simulink model "questao1lcsd3"  (R2026a)
settings: Solver=VariableStepAuto  MaxStep=1e-3
settings Model: Creator=shumy  LastModifiedBy=shumy

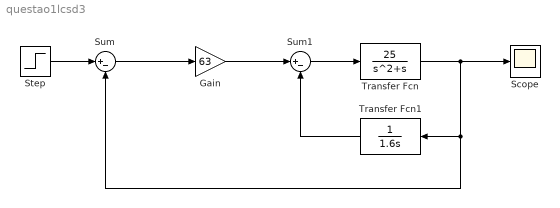
== system questao1lcsd3 ==
  Gain : Gain  Gain=63
  Scope : Scope
      settings: ActiveDisplayYMinimum=-0.2450985660047002  ActiveDisplayYMaximum=2.2058870940423025
  Step : Step  SampleTime=0
  Sum : Sum  Inputs=|+-
  Sum1 : Sum  Inputs=|+-
  Transfer Fcn : TransferFcn  Numerator=[25]  Denominator=[1 1 0]
  Transfer Fcn1 : TransferFcn  Denominator=[1.6 0]
  wires:
  Step/1 -> Sum/1
  Sum/1 -> Gain/1
  Gain/1 -> Sum1/1
  Sum1/1 -> Transfer Fcn/1
  Transfer Fcn/1 -> Transfer Fcn1/1, Sum/2, Scope/1
  Transfer Fcn1/1 -> Sum1/2
